simulink model "CartControl"  (R2023b)
settings: Solver=FixedStepAuto  StartTime=0.0  StopTime=inf  RelTol=1e-3  EnableMultiTasking=on
libraries: raspberrypiCommlib x2
settings Model: ExtModeTrigDuration=2  Creator=Lenovo  LastModifiedBy=Lenovo
settings SolverCC: PositivePriorityOrder=on
settings OptimizationCC: EnhancedBackFolding=on  PassReuseOutputArgsAs=Individual arguments  ZeroExternalMemoryAtStartup=off  ZeroInternalMemoryAtStartup=off  MaxStackSize=64  OptimizeBlockOrder=speed  DifferentSizesBufferReuse=on  OptimizationCustomize=off  EfficientTunableParamExpr=on
settings DebuggingCC: ParameterTunabilityLossMsg=error  UnconnectedInputMsg=warning  UnconnectedOutputMsg=warning  UnconnectedLineMsg=warning
settings HardwareCC: ProdBitPerPointer=32  ProdBitPerSizeT=32  ProdBitPerPtrDiffT=32  ProdLargestAtomicInteger=Long  ProdLargestAtomicFloat=Double  ProdWordSize=32  ProdLongLongMode=on  ProdHWDeviceType=ARM Compatible->ARM Cortex
settings ModelReferenceCC: EnableRefExpFcnMdlSchedulingChecks=on
settings RTWCC: Description=Embedded Coder  SystemTargetFile=ert.tlc  HardwareBoard=Raspberry Pi  TLCOptions="-aInlineSetEventsForThisBaseRateFcn=TLC_FALSE -aSuppressMultiTaskScheduler=TLC_FALSE  -aRateBasedStepFcn=0"  TemplateMakefile=ert_default_tmf  Toolchain=GNU GCC Embedded Linux  BuildConfiguration=Faster Runs  DLArmComputeVersion=19.05
settings CodeAppCC: ForceParamTrailComments=on  IgnoreCustomStorageClasses=off  OperatorAnnotations=on  SimulinkDataObjDesc=on  SFDataObjDesc=on  InsertBlockDesc=on
settings ERTTargetCC: SupportContinuousTime=on  SupportVariableSizeSignals=on  ExtModeTransport=2  ExtModeStaticAlloc=on  ExtModeMexFile=ext_xcp  ExtModeIntrfLevel=Level2 - Open

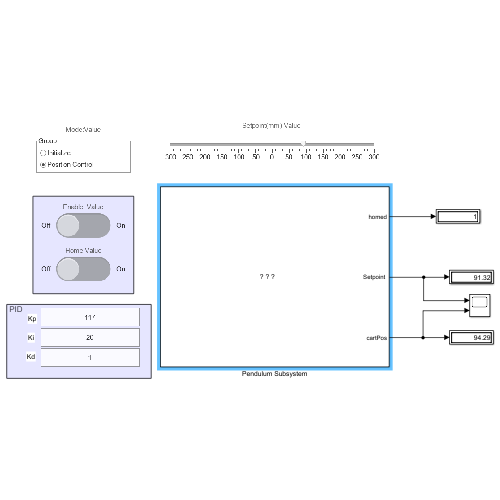
[thumbnail: Simulink's stored preview of the top-level diagram]
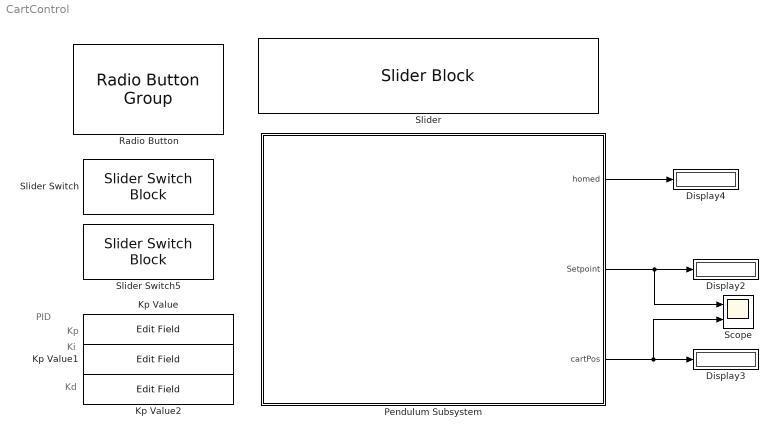
== system CartControl ==
  note: Ki
  note: Kd
  note: Kp
  note: PID
  Display2 : Display
  Display3 : Display
  Display4 : Display
  Kp Value : EditField  LabelPosition=Hide  ShowInitialText=on  Alignment=Center
  Kp Value1 : EditField  LabelPosition=Hide  ShowInitialText=on  Alignment=Center
  Kp Value2 : EditField  LabelPosition=Hide  ShowInitialText=on  Alignment=Center
  Pendulum Subsystem : Subsystem
      mask Display: image('pendulum.png'); % Use "Edit Image" on toolstrip to change.
  Radio Button : RadioButtonGroup  SelectedLabel=Position Control  ButtonGroupName=Group
      settings: Values={{'Initialize', 'Position Control'}, [0 1]}
  Scope : Scope  NumInputPorts=2
  Slider : SliderBlock  ScaleMin=-300  ScaleMax=300  TickInterval=50
  Slider Switch : SliderSwitchBlock
      settings: Values={{'Off', 'On'}, [0 1]}
  Slider Switch5 : SliderSwitchBlock
      settings: Values={{'Off', 'On'}, [0 1]}
  wires:
  Pendulum Subsystem/2("Setpoint ") -> Scope/1, Display2/1
  Pendulum Subsystem/1(homed) -> Display4/1
  Pendulum Subsystem/3(cartPos) -> Scope/2, Display3/1

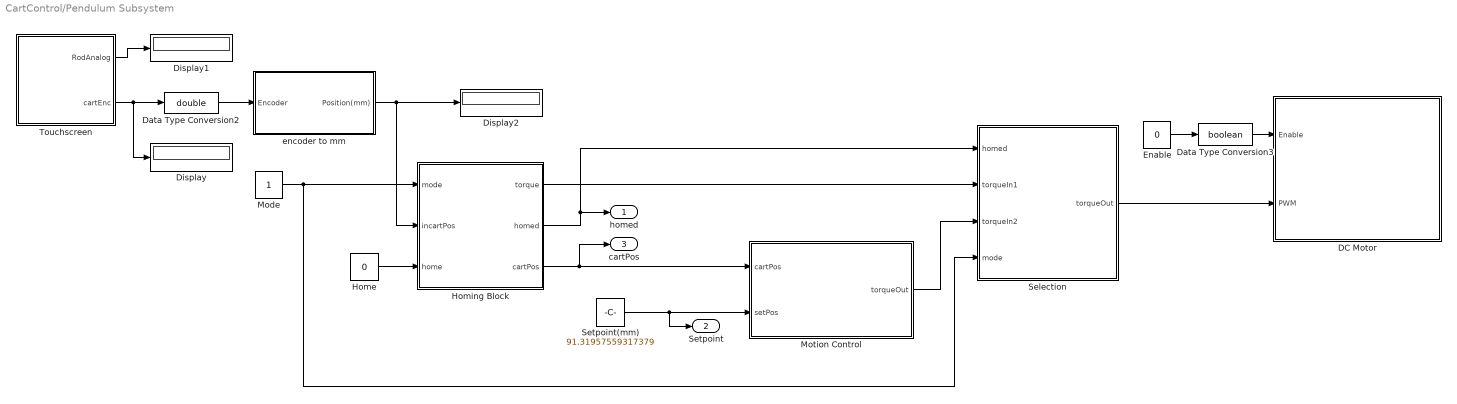
== system CartControl/Pendulum Subsystem ==
  DC Motor : Subsystem
  Data Type Conversion2 : DataTypeConversion  OutDataTypeStr=double  SaturateOnIntegerOverflow=off  RndMeth=Floor
  Data Type Conversion3 : DataTypeConversion  OutDataTypeStr=boolean  SaturateOnIntegerOverflow=off  RndMeth=Floor
  Display : Display
  Display1 : Display
  Display2 : Display
  "Enable " : Constant  Value=0
  Home : Constant  Value=0
  Homing Block : MATLAB Function  TreatAsAtomicUnit=on
  Mode : Constant
  Motion Control : Subsystem
  Selection : MATLAB Function  TreatAsAtomicUnit=on
  Setpoint(mm) : Constant  Value=91.31957559317379  OutMin=[-300]  OutMax=[300]
  Touchscreen : Subsystem
  encoder to mm : Subsystem
  homed : Outport
  "Setpoint " : Outport  Port=2  VectorParamsAs1DForOutWhenUnconnected=off
  cartPos : Outport  Port=3
  wires:
  Touchscreen/2(cartEnc) -> Display/1, Data Type Conversion2/1
  "Enable "/1 -> Data Type Conversion3/1
  Data Type Conversion3/1 -> DC Motor/1(Enable)
  Homing Block/1(torque) -> Selection/2(torqueIn1)
  Homing Block/3(cartPos) -> cartPos/1, Motion Control/1(cartPos)
  Homing Block/2(homed) -> Selection/1(homed), homed/1
  Home/1 -> Homing Block/3(home)
  Mode/1 -> Selection/4(mode), Homing Block/1(mode)
  Motion Control/1(torqueOut) -> Selection/3(torqueIn2)
  Data Type Conversion2/1 -> encoder to mm/1(Encoder)
  encoder to mm/1(Position(mm)) -> Display2/1, Homing Block/2(incartPos)
  Setpoint(mm)/1 -> "Setpoint "/1, Motion Control/2(setPos)
  Touchscreen/1(RodAnalog) -> Display1/1
  Selection/1(torqueOut) -> DC Motor/2(PWM)

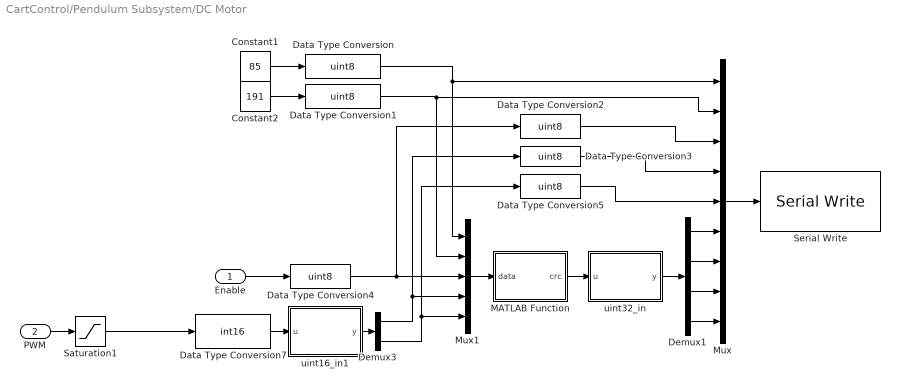
== system CartControl/Pendulum Subsystem/DC Motor ==
  Enable : Inport
  PWM : Inport  Port=2
  Constant1 : Constant  Value=85
  Constant2 : Constant  Value=191
  Data Type Conversion{,1..5} (6 alike) : DataTypeConversion  OutDataTypeStr=uint8  SaturateOnIntegerOverflow=off  RndMeth=Floor
  Data Type Conversion7 : DataTypeConversion  OutDataTypeStr=int16  SaturateOnIntegerOverflow=off  RndMeth=Floor
  Demux1 : Demux
  Demux3 : Demux  Outputs=2
  MATLAB Function : MATLAB Function  TreatAsAtomicUnit=on
  Mux : Mux  Inputs=9
  Mux1 : Mux  Inputs=5
  Saturation1 : Saturate  UpperLimit=1000  LowerLimit=-1000
  Serial Write : raspberrypiCommlib/Serial Write  board=Pi 3 Model B  SCIModule_=/dev/serial0  Baudrate_=115200  Parity=None  StopBits_=1  HardwareFlowControl=None  ByteOrder=LittleEndian  OutputStatus=off  blockPlatform=RaspberryPi
  uint16_in1 : MATLAB Function  TreatAsAtomicUnit=on
  uint32_in : MATLAB Function  TreatAsAtomicUnit=on
  wires:
  Saturation1/1 -> Data Type Conversion7/1
  PWM/1 -> Saturation1/1
  Data Type Conversion4/1 -> Data Type Conversion2/1, Mux1/3
  Demux1/1 -> Mux/6
  Demux1/2 -> Mux/7
  Demux1/3 -> Mux/8
  Demux1/4 -> Mux/9
  Demux3/2 -> Mux1/5, Data Type Conversion5/1
  Constant1/1 -> Data Type Conversion/1
  Constant2/1 -> Data Type Conversion1/1
  Enable/1 -> Data Type Conversion4/1
  Mux1/1 -> MATLAB Function/1(data)
  MATLAB Function/1(crc) -> uint32_in/1(u)
  uint32_in/1(y) -> Demux1/1
  Data Type Conversion2/1 -> Mux/3
  Mux/1 -> Serial Write/1
  Data Type Conversion1/1 -> Mux1/2, Mux/2
  Data Type Conversion3/1 -> Mux/4
  Data Type Conversion/1 -> Mux1/1, Mux/1
  Demux3/1 -> Mux1/4, Data Type Conversion3/1
  Data Type Conversion5/1 -> Mux/5
  uint16_in1/1(y) -> Demux3/1
  Data Type Conversion7/1 -> uint16_in1/1(u)

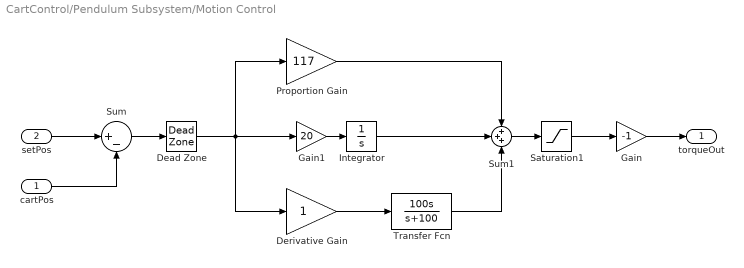
== system CartControl/Pendulum Subsystem/Motion Control ==
  cartPos : Inport
  setPos : Inport  Port=2
  Dead Zone : DeadZone  LowerValue=-1  UpperValue=1
  Derivative Gain : Gain
  Gain : Gain  Gain=-1
  Gain1 : Gain  Gain=20
  Integrator : Integrator  LimitOutput=on  UpperSaturationLimit=350  LowerSaturationLimit=-350
  Proportion Gain : Gain  Gain=117
  Saturation1 : Saturate  UpperLimit=1500  LowerLimit=-1500
  Sum : Sum  Inputs=|+-
  Sum1 : Sum  Inputs=+++
  Transfer Fcn : TransferFcn  Numerator=[100 0]  Denominator=[1 100]
  torqueOut : Outport
  wires:
  setPos/1 -> Sum/1
  cartPos/1 -> Sum/2
  Sum/1 -> Dead Zone/1
  Gain/1 -> torqueOut/1
  Saturation1/1 -> Gain/1
  Gain1/1 -> Integrator/1
  Integrator/1 -> Sum1/2
  Derivative Gain/1 -> Transfer Fcn/1
  Proportion Gain/1 -> Sum1/1
  Dead Zone/1 -> Proportion Gain/1, Gain1/1, Derivative Gain/1
  Sum1/1 -> Saturation1/1
  Transfer Fcn/1 -> Sum1/3

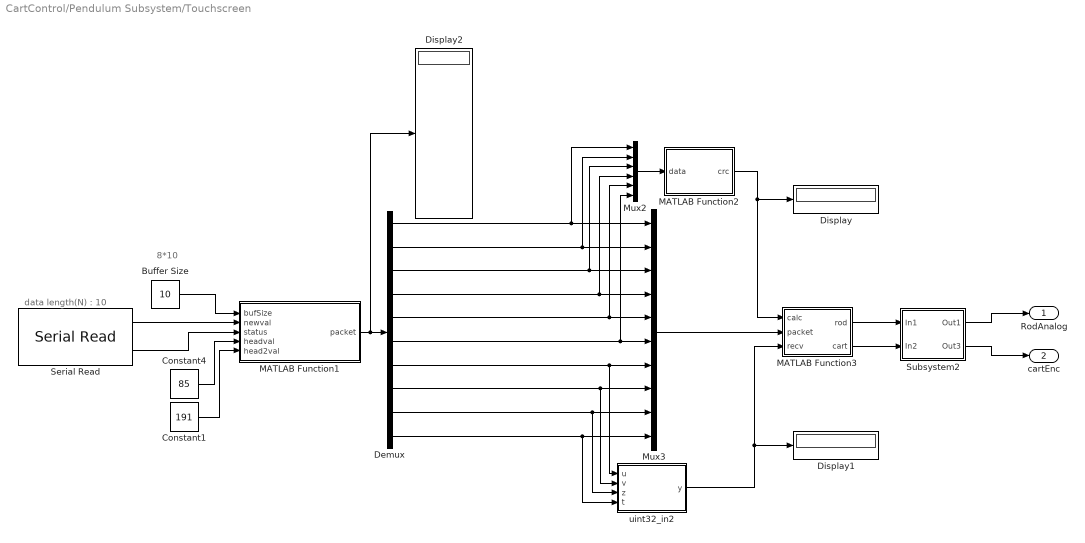
== system CartControl/Pendulum Subsystem/Touchscreen ==
  note: data length(N) : 10
  note: 8*10
  Buffer Size : Constant  Value=10  OutDataTypeStr=uint8
  Constant1 : Constant  Value=191  OutDataTypeStr=uint8
  Constant4 : Constant  Value=85  OutDataTypeStr=uint8
  Demux : Demux  Outputs=10
  Display : Display
  Display1 : Display
  Display2 : Display
  MATLAB Function1 : MATLAB Function  TreatAsAtomicUnit=on
  MATLAB Function2 : MATLAB Function  TreatAsAtomicUnit=on
  MATLAB Function3 : MATLAB Function  TreatAsAtomicUnit=on
  Mux2 : Mux  Inputs=6
  Mux3 : Mux  Inputs=10
  Serial Read : raspberrypiCommlib/Serial Read  board=Pi 3 Model B  SCIModule_=/dev/serial0  Baudrate_=115200  Parity=None  StopBits_=1  HardwareFlowControl=None  ByteOrder=LittleEndian  DataLength=10  DataType=uint8  OutputStatus=on  SampleTime=0.004  blockPlatform=RaspberryPi
  Subsystem2 : Subsystem
  uint32_in2 : MATLAB Function  TreatAsAtomicUnit=on
  RodAnalog : Outport
  cartEnc : Outport  Port=2
  wires:
  Demux/1 -> Mux3/1, Mux2/1
  Demux/6 -> Mux3/6, Mux2/6
  Subsystem2/1(Out1) -> RodAnalog/1
  Mux2/1 -> MATLAB Function2/1(data)
  Constant1/1 -> MATLAB Function1/5(head2val)
  MATLAB Function3/2(cart) -> Subsystem2/2(In2)
  Demux/4 -> Mux3/4, Mux2/4
  Demux/10 -> Mux3/10, uint32_in2/4(t)
  Demux/3 -> Mux3/3, Mux2/3
  uint32_in2/1(y) -> Display1/1, MATLAB Function3/3(recv)
  Demux/8 -> Mux3/8, uint32_in2/2(v)
  Buffer Size/1 -> MATLAB Function1/1(bufSize)
  Demux/5 -> Mux3/5, Mux2/5
  Demux/2 -> Mux3/2, Mux2/2
  Constant4/1 -> MATLAB Function1/4(headval)
  Serial Read/2 -> MATLAB Function1/3(status)
  Mux3/1 -> MATLAB Function3/2(packet)
  MATLAB Function2/1(crc) -> Display/1, MATLAB Function3/1(calc)
  MATLAB Function1/1(packet) -> Display2/1, Demux/1
  Demux/7 -> Mux3/7, uint32_in2/1(u)
  Subsystem2/2(Out3) -> cartEnc/1
  MATLAB Function3/1(rod) -> Subsystem2/1(In1)
  Demux/9 -> Mux3/9, uint32_in2/3(z)
  Serial Read/1 -> MATLAB Function1/2(newval)

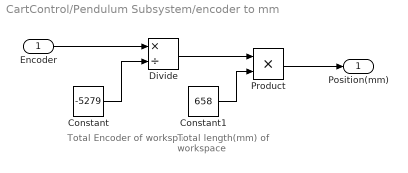
== system CartControl/Pendulum Subsystem/encoder to mm ==
  note: Total Encoder
      | of workspace
  note: Total length(mm)
      | of workspace
  Encoder : Inport
  Constant : Constant  Value=-5279
  Constant1 : Constant  Value=658
  Divide : Product  Inputs=*/
  Product : Product
  Position(mm) : Outport  VectorParamsAs1DForOutWhenUnconnected=off
  wires:
  Encoder/1 -> Divide/1
  Constant/1 -> Divide/2
  Divide/1 -> Product/1
  Constant1/1 -> Product/2
  Product/1 -> Position(mm)/1

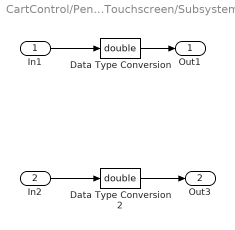
== system CartControl/Pendulum Subsystem/Touchscreen/Subsystem2 ==
  In1 : Inport
  In2 : Inport  Port=2
  Data Type Conversion : DataTypeConversion  OutDataTypeStr=double  SaturateOnIntegerOverflow=off  RndMeth=Floor
  Data Type Conversion2 : DataTypeConversion  OutDataTypeStr=double  SaturateOnIntegerOverflow=off  RndMeth=Floor
  Out1 : Outport
  Out3 : Outport  Port=2
  wires:
  Data Type Conversion2/1 -> Out3/1
  Data Type Conversion/1 -> Out1/1
  In2/1 -> Data Type Conversion2/1
  In1/1 -> Data Type Conversion/1

== matlab function CartControl/Pendulum Subsystem/Selection ==
  settings: updateMethod=DISCRETE
  data: homed input; torqueIn1 input; torqueOut output; torqueIn2 input; mode input
function torqueOut  =fcn(homed,torqueIn1,torqueIn2,mode)
persistent torqueval

if isempty(torqueval)
    torqueval=0;
end

if (mode==0)
    torqueval=-torqueIn1;
end
if (mode==1)
    if (homed==1)
            torqueval=-torqueIn2;
        else
            torqueval=0;
    end
end
torqueOut=torqueval;
end

== matlab function CartControl/Pendulum Subsystem/Homing Block ==
  settings: updateMethod=DISCRETE
  data: torque output; mode input; incartPos input; home input; homed output; cartPos output
function [torque,homed,cartPos]=fcn(mode,incartPos,home)
persistent torqueval
persistent state
persistent precartEnc
persistent homeval
persistent counter
persistent i
persistent precart
persistent prepos
persistent precartArray

if isempty(state)
    torqueval=0;
    state=0;
    precartEnc=0;
    precartArray=[0 0 0 0 0 0 0 0 0 0];
    homeval=0;
    counter=0;
    i=0;
    precart=0;
    prepos=0;
end

if (mode==0)
    if (homeval==0)
        if (home==0)
            state=0;
            homeval=0;
            counter=0;
            precart=0;
            prepos=0;
            precartArray=[0 0 0 0 0 0 0 0 0 0];
        end
        if (state==0)
            torqueval=0;
            if (home==1)
                state=1;
            end
        elseif (state==1)
            torqueval=500;
            state=2;
        elseif (state==2) % 4 sec wait and check final cartpos
            if (counter==100)
                if (all(precartArray==incartPos))
                    torqueval=0;
                    homeval=1;
                    prepos=incartPos;
                else
                      i=i+1;
                      precartArray(i)=precart;
                      if (i==10)
                          i=0;
                      end             
                      precart=incartPos;
                end
            else
                counter=counter+1;
            end
        end
    else
        if (home==0)
            state=0;
            homeval=0;
            counter=0;
            precartEnc=0;
            prepos=0;
        end
    end
end
homed=homeval;
torque=torqueval;
if (homed==1)
    precartEnc=-329-prepos;
    cartPos=precartEnc+incartPos;
else
    cartPos=incartPos;
end
end

== matlab function CartControl/Pendulum Subsystem/DC Motor/MATLAB Function ==
  data: data input; crc output
function crc = crc_32(data)

% Computes the CRC-32/MPEG-2 checksum value of a byte vector.
% Uses a left shifting (not reflected) CRC along with the 
% CRC polynomial 0x04C11DB7 and initial CRC value of 0xFFFFFFFF,
% and is not post complemented.
%--------------------------------------------------------------------------
%   Version:    130
%   Programmer: Oliver Calderbank
%   Date:       21-07-2019

% Initialize variables
crc  = uint32(hex2dec('FFFFFFFF'));
poly = uint32(hex2dec('04C11DB7'));
data = uint8(data);
temp = uint32(data);

for i = 1:length(data)
    % xor next byte to upper bits of crc
    crc = bitxor(crc,uint32(bitshift(temp(i),24)));
    for j = 1:8
        msb = bitsra(crc,31);
        crc = bitsll(crc,1);
        if msb == 1 
            crc = bitxor(crc,poly);
        end 
    end
end
end

== matlab function CartControl/Pendulum Subsystem/DC Motor/uint16_in1 ==
  data: u input; y output
function y = fcn(u)
t=typecast(int16(u),'uint8');
y = [t(1) t(2)];

== matlab function CartControl/Pendulum Subsystem/DC Motor/uint32_in ==
  data: u input; y output
function y = fcn(u)
t=typecast(uint32(u),'uint8');
y = [t(1) t(2) t(3) t(4)];

== matlab function CartControl/Pendulum Subsystem/Touchscreen/MATLAB Function1 ==
  settings: updateMethod=DISCRETE
  data: bufSize input uint8 size=1; newval input uint8 size=10; status input; headval input uint8; packet output size=10; head2val input
function packet   = fcn(bufSize,newval,status,headval,head2val)
%initializing
persistent val;
persistent bff;
persistent packetindex
if isempty(bff)
    packetindex =uint8(zeros(1,10));
end
if isempty(val)
    val=0;
    bff = zeros(bufSize,1); %initializing
    inc=0;
else
    inc=1;
end

ind =uint8( mod(val-1,bufSize) + 1); %current index
if isempty(bff)
    bff = zeros(bufSize,1); %initializing
end
if status==0  %UART Status
    for i = 1:1:10
        bff(mod(ind-1+i-1,bufSize)+1) = newval(i); %adding the circular buffer
    end
    if inc==1
        val=val+10;   
    end
end
if ind==0
    val=0;
end
buffout =uint8( bff((1:80)));  % whole buffer
head=uint8(find(bff(ind+1:end)==headval)+double(ind)); %finding first header
if isempty(head)
    head=uint8(find(bff(1:end)==headval));
end
if bff(mod(head(1),bufSize)+1)==head2val %header2 check
    packetindex=[mod(head(1)-1,bufSize)+1 mod(head(1),bufSize)+1 mod(head(1)+1,bufSize)+1 mod(head(1)+2,bufSize)+1 ... %adding correct package's index to array
                 mod(head(1)+3,bufSize)+1 mod(head(1)+4,bufSize)+1 mod(head(1)+5,bufSize)+1 mod(head(1)+6,bufSize)+1 mod(head(1)+7,bufSize)+1 mod(head(1)+8,bufSize)+1];
end
lastadd=uint8(bff(head(1)+1));
packet=bff(packetindex);

== matlab function CartControl/Pendulum Subsystem/Touchscreen/MATLAB Function2 ==
  data: data input; crc output
function crc = crc_32(data)

% Computes the CRC-32/MPEG-2 checksum value of a byte vector.
% Uses a left shifting (not reflected) CRC along with the 
% CRC polynomial 0x04C11DB7 and initial CRC value of 0xFFFFFFFF,
% and is not post complemented.
%--------------------------------------------------------------------------
%   Version:    130
%   Programmer: Oliver Calderbank
%   Date:       21-07-2019

% Initialize variables
crc  = uint32(hex2dec('FFFFFFFF'));
poly = uint32(hex2dec('04C11DB7'));
data = uint8(data);
temp = uint32(data);

for i = 1:length(data)
    % xor next byte to upper bits of crc
    crc = bitxor(crc,uint32(bitshift(temp(i),24)));
    for j = 1:8
        msb = bitsra(crc,31);
        crc = bitsll(crc,1);
        if msb == 1 
            crc = bitxor(crc,poly);
        end 
    end
end
end

== matlab function CartControl/Pendulum Subsystem/Touchscreen/MATLAB Function3 ==
  data: calc input; packet input; rod output int16 size=1; recv input; cart output int16 size=1
function [rod,cart] = fcn(calc,packet,recv)
persistent validpack;
persistent validpack2;
if isempty(validpack)
    Axisx=[packet(3) packet(4)];
    validpack=typecast(uint8(Axisx),'int16');
end
if isempty(validpack2)
    Axisy=[packet(5) packet(6)];
    validpack2=typecast(uint8(Axisy),'int16');
end
if calc==recv
    Axisx=[packet(3) packet(4)];
    validpack=typecast(uint8(Axisx),'int16');
    Axisy=[packet(5) packet(6)];
    validpack2=typecast(uint8(Axisy),'int16');
    rod=validpack;
    cart=validpack2;
else
	rod=validpack;
    cart=validpack2;
end

== matlab function CartControl/Pendulum Subsystem/Touchscreen/uint32_in2 ==
  data: u input; y output uint32 size=1; v input; z input; t input
function y = fcn(u,v,z,t)
x=[u v z t];
k=typecast(uint8(x),'uint32');
y = k;
